simulink model "system2020b"  (R2020b)
settings: Solver=VariableStepAuto  StartTime=0.0  StopTime=50  RelTol=1e-3
InitFcn:
  | parametriEgo
values from neighbouring files (symbols this model uses):
  campnormalized = campmag/sqrt(campmag(1)^2+campmag(2)^2+campmag(3)^2)    [parametriEgo.m]
  g = 9.81    [kalman_jacobian.m]    (also in parametriEgo.m = [0; 0; -9.81])
  initial_conditions = [0,0,0*pi/180,0*pi/180,0,0]    [parametriEgo.m]
  k_e_qf = 0.1    [ego_control_gains_sensors.m]
  ki_e_nu_speed = 2.5    [ego_control_gains_sensors.m]
  kp_e_nu_phidot = 7    [ego_control_gains_sensors.m]
  kp_e_nu_speed = 6    [ego_control_gains_sensors.m]
  kp_e_nu_thetadot = 7    [ego_control_gains_sensors.m]
  kp_e_theta = 40    [ego_control_gains_sensors.m]
  l = 0.248    [parametriEgo.m]
  L = 0.379    [parametriEgo.m]
  mb = 21.7+0.536*10+0.381*2    (= 27.822)    [parametriEgo.m]
  mw = 1.6    [parametriEgo.m]
  P0 = 1500*eye(7)    [parametriEgo.m]
  r = 0.13    [parametriEgo.m]
  seedAcc1 = ceil(rand()*10)    [parametriEgo.m]
  seedAcc2 = ceil(rand()*10)    [parametriEgo.m]
  seedGyro1 = ceil(rand()*10)    [parametriEgo.m]
  seedGyro2 = ceil(rand()*10)    [parametriEgo.m]
  tau_max = 11    [parametriEgo.m]
  totAccNoisePower = (accNoiseDens* 10^-6 * 9.8)^2    (= 8.6436e-06)    [parametriEgo.m]
  totGyroNoisePower = (gyroNoiseDens * pi/180)^2    (= 3.04617419787e-06)    [parametriEgo.m]
  Ts = 1/100    (= 0.01)    [parametriEgo.m]
  TsController = 1/100    (= 0.01)    [parametriEgo.m]
  TsGraph = 1/100    (= 0.01)    [parametriEgo.m]
  x0 = zeros(7,1)    [parametriEgo.m]
undefined symbols (not defined in the file or in its folder): alpha
libraries: simulink_extras x45, simulink x10, eeGeneralControl x3
(part 2 of 3)

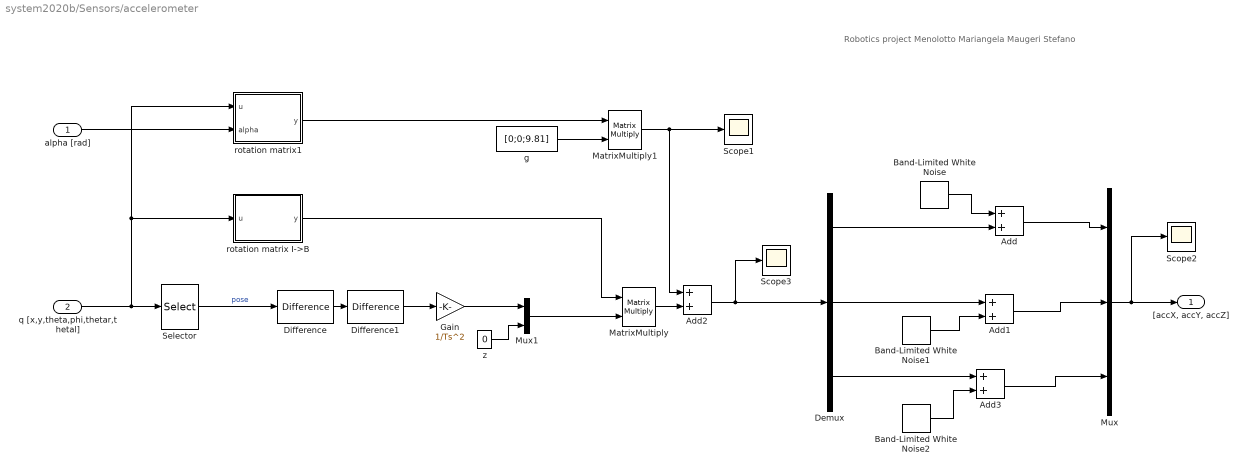
== system system2020b/Sensors/accelerometer ==
  note: Robotics project
      | Menolotto Mariangela
      | Maugeri Stefano
  alpha [rad] : Inport
  q [x,y,theta,phi,thetar,thetal] : Inport  Port=2
  Add{,1..3} (4 alike) : Sum
  Band-Limited White Noise : simulink/Sources/Band-Limited White Noise  Cov=abs(totAccNoisePower)  Ts=0.1  seed=abs(seedAcc1)+1
  Band-Limited White Noise1 : simulink/Sources/Band-Limited White Noise  Cov=totAccNoisePower  Ts=0.1  seed=abs(seedAcc2)+22
  Band-Limited White Noise2 : simulink/Sources/Band-Limited White Noise  Cov=totAccNoisePower  Ts=0.1  seed=abs(seedAcc1+13)
  Demux : Demux  Outputs=3
  Difference : simulink/Discrete/Difference  ICPrevInput=0.0  OutMin=[]  OutMax=[]  OutDataType=fixdt(1, 16)  OutScaling=2^-10  DoSatur=off
  Difference1 : simulink/Discrete/Difference  ICPrevInput=0.0  OutMin=[]  OutMax=[]  OutDataType=fixdt(1, 16)  OutScaling=2^-10  DoSatur=off
  Gain : Gain  Gain=1/Ts^2
  MatrixMultiply : Product  Multiplication=Matrix(*)
  MatrixMultiply1 : Product  Multiplication=Matrix(*)
  Mux : Mux  Inputs=3
  Mux1 : Mux  Inputs=2
  Scope1 : Scope
  Scope2 : Scope
  Scope3 : Scope
  Selector : Selector  InputPortWidth=6  IndexOptions=Index vector (dialog)  Indices=[1 2]  OutputSizes=1
  g : Constant  Value=[0;0;9.81]
  rotation matrix I->B : MATLAB Function  TreatAsAtomicUnit=on
  rotation matrix1 : MATLAB Function  TreatAsAtomicUnit=on
  z : Constant  Value=0
  "[accX, accY, accZ]" : Outport
  wires:
  q [x,y,theta,phi,thetar,thetal]/1 -> rotation matrix I->B/1(u), rotation matrix1/1(u), Selector/1
  Selector/1 -> Difference/1  "pose"
  Demux/1 -> Add/2
  Demux/2 -> Add1/1
  Band-Limited White Noise1/1 -> Add1/2
  Band-Limited White Noise/1 -> Add/1
  Mux/1 -> Scope2/1, "[accX, accY, accZ]"/1
  Add1/1 -> Mux/2
  Add/1 -> Mux/1
  z/1 -> Mux1/2
  Mux1/1 -> MatrixMultiply/2
  rotation matrix I->B/1(y) -> MatrixMultiply/1
  MatrixMultiply/1 -> Add2/2
  rotation matrix1/1(y) -> MatrixMultiply1/1
  g/1 -> MatrixMultiply1/2
  Add2/1 -> Scope3/1, Demux/1
  MatrixMultiply1/1 -> Add2/1, Scope1/1
  Demux/3 -> Add3/1
  Band-Limited White Noise2/1 -> Add3/2
  Add3/1 -> Mux/3
  alpha [rad]/1 -> rotation matrix1/2(alpha)
  Difference/1 -> Difference1/1
  Difference1/1 -> Gain/1
  Gain/1 -> Mux1/1

== system system2020b/Sensors/encoder ==
  note: Robotics project
      | Menolotto Mariangela
      | Maugeri Stefano
  q [x,y,theta,phi,thetar,thetal] : Inport
  Demux : Demux  Outputs=2
  Mux : Mux  Inputs=2
  Random Number : RandomNumber  Variance=0.03/3  SampleTime=0.1
  Random Number1 : RandomNumber  Variance=0.03/3  SampleTime=0.1
  Selector : Selector  InputPortWidth=6  IndexOptions=Index vector (dialog)  Indices=[5 6]  OutputSizes=1
  Sum : Sum  Inputs=++|
  Sum1 : Sum  Inputs=|++
  "thetar, thetal" : Outport
  wires:
  q [x,y,theta,phi,thetar,thetal]/1 -> Selector/1
  Selector/1 -> Demux/1
  Mux/1 -> "thetar, thetal"/1
  Sum/1 -> Mux/1
  Demux/1 -> Sum/2
  Sum1/1 -> Mux/2
  Demux/2 -> Sum1/1
  Random Number1/1 -> ?
  Random Number/1 -> ?

== system system2020b/Sensors/gyroscope ==
  note: Robotics project
      | Menolotto Mariangela
      | Maugeri Stefano
  "nu [v_avaz, theta dot, phi dot]" : Inport
  q [x,y,theta,phi,thetar,thetal] : Inport  Port=2
  Add : Sum
  Add1 : Sum
  Add2 : Sum
  Band-Limited White Noise : simulink/Sources/Band-Limited White Noise  Cov=totGyroNoisePower  Ts=0.1  seed=seedGyro1
  Band-Limited White Noise1 : simulink/Sources/Band-Limited White Noise  Cov=totGyroNoisePower  Ts=0.1  seed=seedGyro2+1
  Band-Limited White Noise2 : simulink/Sources/Band-Limited White Noise  Cov=totGyroNoisePower  Ts=0.1  seed=seedGyro1-2
  Demux : Demux  Outputs=3
  MATLAB Function : MATLAB Function  TreatAsAtomicUnit=on
  Mux : Mux  Inputs=3
  Radians to Degrees : simulink_extras/Transformations/Radians to Degrees
  Scope : Scope
  Scope1 : Scope
  Selector : Selector  InputPortWidth=3  IndexOptions=Index vector (dialog)  Indices=[2 3]  OutputSizes=1
  omega_c hat : Outport
  wires:
  "nu [v_avaz, theta dot, phi dot]"/1 -> Selector/1
  Selector/1 -> MATLAB Function/1(u)  "theta dot, phi dot"
  Demux/1 -> Add/2
  Demux/3 -> Add1/1
  Mux/1 -> Scope/1, omega_c hat/1
  Band-Limited White Noise/1 -> Add/1
  Band-Limited White Noise1/1 -> Add1/2
  Add/1 -> Mux/1
  Add1/1 -> Mux/3
  Add2/1 -> Mux/2
  MATLAB Function/1(omegac) -> Radians to Degrees/1, Demux/1
  q [x,y,theta,phi,thetar,thetal]/1 -> MATLAB Function/2(q)
  Demux/2 -> Add2/2
  Band-Limited White Noise2/1 -> Add2/1
  Radians to Degrees/1 -> Scope1/1

== system system2020b/Sensors/magnetometer    ==
  note: Robotics project
      | Menolotto Mariangela
      | Maugeri Stefano
  alpha [rad] : Inport
  q [x,y,theta,phi,thetar,thetal] : Inport  Port=2
  Add : Sum
  Band-Limited White Noise : simulink/Sources/Band-Limited White Noise  Cov=abs(totGyroNoisePower)  Ts=0.1  seed=seedGyro1
  MATLAB Function : MATLAB Function  TreatAsAtomicUnit=on
  magnetometer : Outport
  wires:
  MATLAB Function/1(y) -> Add/2
  alpha [rad]/1 -> MATLAB Function/1(alpha)
  q [x,y,theta,phi,thetar,thetal]/1 -> MATLAB Function/2(q)
  Band-Limited White Noise/1 -> Add/1
  Add/1 -> magnetometer/1

== system system2020b/Sensors/mux signals ==
  note: Robotics project
      | Menolotto Mariangela
      | Maugeri Stefano
  q [x,y,theta,phi,thetar,thetal] : Inport
  "nu [v_avaz, theta dot, phi dot]" : Inport  Port=2
  q_dot : Inport  Port=3
  Mux : Mux  Inputs=3
  "[q;nu]" : Outport
  wires:
  q [x,y,theta,phi,thetar,thetal]/1 -> Mux/1
  "nu [v_avaz, theta dot, phi dot]"/1 -> Mux/2
  Mux/1 -> "[q;nu]"/1
  q_dot/1 -> Mux/3

== system system2020b/Sensors/range finder ==
  note: Robotics project
      | Menolotto Mariangela
      | Maugeri Stefano
  q : Inport
  MATLAB Function1 : MATLAB Function  TreatAsAtomicUnit=on
  Quantizer : Quantizer  QuantizationInterval=0.001
  Quantizer1 : Quantizer  QuantizationInterval=0.001
  Random Number : RandomNumber  Variance=0.0000001  SampleTime=1/10
  Scope : Scope  NumInputPorts=2
  Scope1 : Scope
  Sum : Sum  Inputs=|++
  distance from ground : Outport
  wires:
  q/1 -> MATLAB Function1/1(q)  "[x,y,theta,phi,thetar,thetal]"
  MATLAB Function1/1(d) -> Scope/1, Sum/1  "new"
  Random Number/1 -> Sum/2, Scope1/1
  Sum/1 -> Quantizer/1, Quantizer1/1
  Quantizer/1 -> Scope/2
  Quantizer1/1 -> distance from ground/1

== system system2020b/Filtering/Kalman filter/store on workspace ==
  note: Robotics project
      | Menolotto Mariangela
      | Maugeri Stefano
  "[v_avanz real, thetadot, phidot] est" : Inport
  "[alpha, theta, phi] est" : Inport  Port=2
  Demux : Demux  Outputs=3
  Demux1 : Demux  Outputs=3
  Radians to Degrees : simulink_extras/Transformations/Radians to Degrees
  Radians to Degrees1 : simulink_extras/Transformations/Radians to Degrees
  Terminator : Terminator
  To Workspace : ToWorkspace  VariableName=thetadot_esimt_kalman  SaveFormat=Timeseries  SampleTime=TsGraph
  To Workspace1 : ToWorkspace  VariableName=phidot_esimt_kamlan  SaveFormat=Timeseries  SampleTime=TsGraph
  To Workspace2 : ToWorkspace  VariableName=alpha_esimt_kalman  SaveFormat=Timeseries  SampleTime=TsGraph
  To Workspace3 : ToWorkspace  VariableName=theta_esimt_kalman  SaveFormat=Timeseries  SampleTime=TsGraph
  To Workspace4 : ToWorkspace  VariableName=phi_esimt_kalman  SaveFormat=Timeseries  SampleTime=TsGraph
  wires:
  "[v_avanz real, thetadot, phidot] est"/1 -> Radians to Degrees/1
  "[alpha, theta, phi] est"/1 -> Radians to Degrees1/1
  Demux/1 -> Terminator/1
  Demux/2 -> To Workspace/1
  Demux/3 -> To Workspace1/1
  Demux1/1 -> To Workspace2/1
  Demux1/2 -> To Workspace3/1
  Demux1/3 -> To Workspace4/1
  Radians to Degrees/1 -> Demux/1
  Radians to Degrees1/1 -> Demux1/1

== system system2020b/Filtering/Mahony + distance sensor/mahony  with quaternions ==
  note: [v_avanz real, thetadot, phidot] est
  note: Robotics project
      | Menolotto Mariangela
      | Maugeri Stefano
  alpha real [rad] : Inport
  distance from ground : Inport  Port=2
  magnetometro : Inport  Port=3
  "[accX, accY, accZ] with noise" : Inport  Port=4
  omega_c hat with noise : Inport  Port=5
  "[q; nu; q_dot] real" : Inport  Port=6
  MATLAB Function : MATLAB Function  TreatAsAtomicUnit=on
  Manual Switch : ManualSwitch  CurrentSetting=0
  Mux1 : Mux  Inputs=3
  Radians to Degrees : simulink_extras/Transformations/Radians to Degrees
  Scope : Scope
  Selector : Selector  InputPortWidth=3  IndexOptions=Index vector (dialog)  Indices=3  OutputSizes=1
  Zero-Order Hold1 : ZeroOrderHold  SampleTime=Ts
  get phi : MATLAB Function  Commented=on  TreatAsAtomicUnit=on
  get phi1 : MATLAB Function  TreatAsAtomicUnit=on
  mahony filter qith quat : Subsystem
  mux signals : Subsystem
  scope differences (mahony) con quaternioni : Subsystem
  nu est : Outport
  "[q;nu] real" : Outport  Port=2
  "[alpha, theta, phi] est" : Outport  Port=3
  wires:
  "[accX, accY, accZ] with noise"/1 -> mahony filter qith quat/2("[accX, accY, accZ]")
  "[q; nu; q_dot] real"/1 -> mux signals/1("[q; nu; q_dot] real")
  Mux1/1 -> Zero-Order Hold1/1
  omega_c hat with noise/1 -> MATLAB Function/1(omega_c), mahony filter qith quat/3(omega_c hat with noise)
  magnetometro/1 -> mahony filter qith quat/4(magnetometro)
  mux signals/2("[q;nu]") -> "[q;nu] real"/1, scope differences (mahony) con quaternioni/3("[q;nu] real")
  alpha real [rad]/1 -> scope differences (mahony) con quaternioni/4(real alpha)
  get phi/1(phi_star) -> Manual Switch/1
  MATLAB Function/1(thetadot) -> Mux1/2  "theta dot"
  MATLAB Function/2(phidot) -> Mux1/3
  Zero-Order Hold1/1 -> nu est/1, scope differences (mahony) con quaternioni/1(nu est)
  mahony filter qith quat/1("[alpha, theta, phi] est") -> scope differences (mahony) con quaternioni/2("[alpha, theta, phi] est"), "[alpha, theta, phi] est"/1, Selector/1  "[alpha theta phi] est"
  Selector/1 -> MATLAB Function/2(phi)  "phi"
  mux signals/1(v_avanz) -> Mux1/1
  distance from ground/1 -> get phi/1(d), get phi1/1(d)
  Manual Switch/1 -> Radians to Degrees/1, mahony filter qith quat/1(phi_star)
  get phi1/1(phi_star) -> Manual Switch/2
  Radians to Degrees/1 -> Scope/1

== system system2020b/Filtering/Mahony + distance sensor/mahony filter ==
  note: Robotics project
      | Menolotto Mariangela
      | Maugeri Stefano
  phi_star : Inport
  "[accX, accY, accZ]" : Inport  Port=2
  omega_c hat with noise : Inport  Port=3
  magnetometro : Inport  Port=4
  Clock : Clock
  Delay : Delay  DelayLength=1  InitialCondition=eye(3)  SampleTime=Ts
  Delay1 : Delay  DelayLength=1  InitialCondition=[0;0;0]  SampleTime=Ts
  Delay2 : Delay  DelayLength=1  SampleTime=Ts
  MATLAB Function : MATLAB Function  TreatAsAtomicUnit=on
  Mux2 : Mux  Inputs=3
  Zero-Order Hold4 : ZeroOrderHold  SampleTime=Ts
  "get angles " : MATLAB Function  TreatAsAtomicUnit=on
  "[alpha, theta, phi] est" : Outport
  wires:
  MATLAB Function/1(R) -> "get angles "/1(R), Delay/1  "R"
  Delay/1 -> MATLAB Function/4(Rprev)
  MATLAB Function/2(I) -> Delay1/1
  Delay1/1 -> MATLAB Function/5(Iprev)
  "[accX, accY, accZ]"/1 -> MATLAB Function/1(acc)
  omega_c hat with noise/1 -> MATLAB Function/2(gyro)
  magnetometro/1 -> MATLAB Function/3(mb)
  phi_star/1 -> "get angles "/2(phi_star)
  "get angles "/1(alpha) -> Mux2/1
  "get angles "/3(phi) -> Mux2/3
  "get angles "/2(theta) -> Delay2/1, Mux2/2
  Delay2/1 -> "get angles "/4(old_theta)
  Mux2/1 -> "[alpha, theta, phi] est"/1  "angles est"
  Clock/1 -> Zero-Order Hold4/1
  Zero-Order Hold4/1 -> "get angles "/3(t)

== system system2020b/Filtering/Mahony + distance sensor/store on workspace ==
  note: Robotics project
      | Menolotto Mariangela
      | Maugeri Stefano
  "[v_avanz real, thetadot, phidot] est" : Inport
  "[alpha, theta, phi] est" : Inport  Port=2
  Demux : Demux  Outputs=3
  Demux1 : Demux  Outputs=3
  Radians to Degrees : simulink_extras/Transformations/Radians to Degrees
  Radians to Degrees1 : simulink_extras/Transformations/Radians to Degrees
  Terminator : Terminator
  To Workspace : ToWorkspace  VariableName=thetadot_esimt_mahony  SaveFormat=Timeseries  SampleTime=TsGraph
  To Workspace1 : ToWorkspace  VariableName=phidot_esimt_mahony  SaveFormat=Timeseries  SampleTime=TsGraph
  To Workspace2 : ToWorkspace  VariableName=alpha_esimt_mahony  SaveFormat=Timeseries  SampleTime=TsGraph
  To Workspace3 : ToWorkspace  VariableName=theta_esimt_mahony  SaveFormat=Timeseries  SampleTime=TsGraph
  To Workspace4 : ToWorkspace  VariableName=phi_esimt_mahony  SaveFormat=Timeseries  SampleTime=TsGraph
  wires:
  "[v_avanz real, thetadot, phidot] est"/1 -> Radians to Degrees/1
  "[alpha, theta, phi] est"/1 -> Radians to Degrees1/1
  Demux/1 -> Terminator/1
  Demux/2 -> To Workspace/1
  Demux/3 -> To Workspace1/1
  Demux1/1 -> To Workspace2/1
  Demux1/2 -> To Workspace3/1
  Demux1/3 -> To Workspace4/1
  Radians to Degrees/1 -> Demux/1
  Radians to Degrees1/1 -> Demux1/1

== system system2020b/Physical system/old model/LQR con linearizzato ==
  note: Robotics project
      | Menolotto Mariangela
      | Maugeri Stefano
  q : Inport
  nu : Inport  Port=2
  Gain : Gain  Gain=-1
  Integrator : Integrator
  LQR : MATLAB Function  TreatAsAtomicUnit=on
  MATLAB Function1 : MATLAB Function  TreatAsAtomicUnit=on
  MATLAB Function2 : MATLAB Function  TreatAsAtomicUnit=on
  MatrixMultiply : Product  Multiplication=Matrix(*)
  Mux : Mux  Inputs=3
  Saturation : Saturate  UpperLimit=tau_max  LowerLimit=-tau_max
  Selector : Selector  InputPortWidth=6  IndexOptions=Index vector (dialog)  Indices=[3 4]  OutputSizes=1
  Selector1 : Selector  InputPortWidth=3  IndexOptions=Index vector (dialog)  Indices=1  OutputSizes=1
  To Workspace1 : ToWorkspace  VariableName=nu1_int  SaveFormat=Timeseries  SampleTime=TsGraph
  tau : Outport
  wires:
  MATLAB Function1/1(B_ss_numerica) -> LQR/2(B_ss)
  LQR/1(K) -> Gain/1
  MATLAB Function2/1(A_ss_numerica) -> LQR/1(A_ss)
  Gain/1 -> MatrixMultiply/1
  MatrixMultiply/1 -> Saturation/1  "u = - Kx"
  nu/1 -> Selector1/1, Mux/1
  q/1 -> Selector/1
  Mux/1 -> MatrixMultiply/2
  Selector/1 -> Mux/3
  Saturation/1 -> tau/1  "nu"
  Selector1/1 -> Integrator/1
  Integrator/1 -> Mux/2, To Workspace1/1

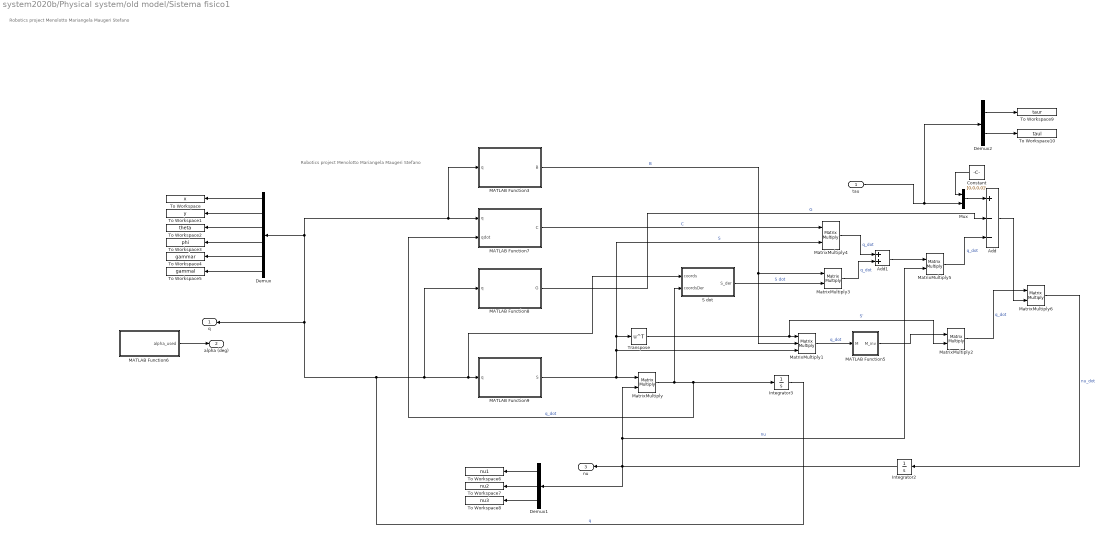
== system system2020b/Physical system/old model/Sistema fisico1 ==
  note: Robotics project
      | Menolotto Mariangela
      | Maugeri Stefano
  note: Robotics project
      | Menolotto Mariangela
      | Maugeri Stefano
  tau : Inport
  Add : Sum  Inputs=+--
  Add1 : Sum
  Constant : Constant  Value=[0,0,0,0]'
  Demux : Demux  Outputs=6
  Demux1 : Demux  Outputs=3
  Demux2 : Demux  Outputs=2
  Integrator2 : Integrator  InitialCondition=[0; 0; 0]
  Integrator3 : Integrator  InitialCondition=initial_conditions
  MATLAB Function3 : MATLAB Function  TreatAsAtomicUnit=on
  MATLAB Function5 : MATLAB Function  TreatAsAtomicUnit=on
  MATLAB Function6 : MATLAB Function  TreatAsAtomicUnit=on
  MATLAB Function7 : MATLAB Function  TreatAsAtomicUnit=on
  MATLAB Function8 : MATLAB Function  TreatAsAtomicUnit=on
  MATLAB Function9 : MATLAB Function  TreatAsAtomicUnit=on
  MatrixMultiply{,2..6} (6 alike) : Product  Multiplication=Matrix(*)
  MatrixMultiply1 : Product  Inputs=3  Multiplication=Matrix(*)
  Mux : Mux  Inputs=2
  S dot : MATLAB Function  TreatAsAtomicUnit=on
  To Workspace : ToWorkspace  VariableName=x  SaveFormat=Timeseries  SampleTime=TsGraph
  To Workspace1 : ToWorkspace  VariableName=y  SaveFormat=Timeseries  SampleTime=TsGraph
  To Workspace10 : ToWorkspace  VariableName=taul  SaveFormat=Timeseries  SampleTime=TsGraph
  To Workspace2 : ToWorkspace  VariableName=theta  SaveFormat=Timeseries  SampleTime=TsGraph
  To Workspace3 : ToWorkspace  VariableName=phi  SaveFormat=Timeseries  SampleTime=TsGraph
  To Workspace4 : ToWorkspace  VariableName=gammar  SaveFormat=Timeseries  SampleTime=TsGraph
  To Workspace5 : ToWorkspace  VariableName=gammal  SaveFormat=Timeseries  SampleTime=TsGraph
  To Workspace6 : ToWorkspace  VariableName=nu1  SaveFormat=Timeseries  SampleTime=TsGraph
  To Workspace7 : ToWorkspace  VariableName=nu2  SaveFormat=Timeseries  SampleTime=TsGraph
  To Workspace8 : ToWorkspace  VariableName=nu3  SaveFormat=Timeseries  SampleTime=TsGraph
  To Workspace9 : ToWorkspace  VariableName=taur  SaveFormat=Timeseries  SampleTime=TsGraph
  Transpose : Math  Operator=transpose  SaturateOnIntegerOverflow=on
  q : Outport
  alpha (deg) : Outport  Port=2
  nu : Outport  Port=3
  wires:
  MATLAB Function9/1(S) -> MatrixMultiply1/3, Transpose/1, MatrixMultiply4/2, MatrixMultiply/1  "S"
  Integrator3/1 -> MATLAB Function3/1(q), MATLAB Function7/1(q), Demux/1, q/1, MATLAB Function8/1(q), MATLAB Function9/1(q), S dot/1(coords)  "q"
  S dot/1(S_der) -> MatrixMultiply3/2  "S dot"
  MATLAB Function3/1(B) -> MatrixMultiply3/1, MatrixMultiply1/2  "B"
  Integrator2/1 -> Demux1/1, MatrixMultiply5/2, MatrixMultiply/2, nu/1  "nu"
  MATLAB Function8/1(G) -> Add/2  "G"
  Transpose/1 -> MatrixMultiply2/2, MatrixMultiply1/1  "S'"
  MatrixMultiply1/1 -> MATLAB Function5/1(M)  "q_dot"
  MatrixMultiply3/1 -> Add1/2  "q_dot"
  MatrixMultiply/1 -> MATLAB Function7/2(qdot), Integrator3/1, S dot/2(coordsDer)  "q_dot"
  MATLAB Function7/1(C) -> MatrixMultiply4/1  "C"
  Add1/1 -> MatrixMultiply5/1
  MatrixMultiply4/1 -> Add1/1  "q_dot"
  MatrixMultiply5/1 -> Add/3  "q_dot"
  Add/1 -> MatrixMultiply6/2
  MatrixMultiply6/1 -> Integrator2/1  "nu_dot"
  MATLAB Function5/1(M_inv) -> MatrixMultiply2/1
  MatrixMultiply2/1 -> MatrixMultiply6/1  "q_dot"
  MATLAB Function6/1(alpha_used) -> alpha (deg)/1
  Demux/5 -> To Workspace4/1
  Demux/2 -> To Workspace1/1
  Demux/1 -> To Workspace/1
  Demux/3 -> To Workspace2/1
  Demux/4 -> To Workspace3/1
  Demux/6 -> To Workspace5/1
  Mux/1 -> Add/1
  Constant/1 -> Mux/1
  Demux1/1 -> To Workspace6/1
  Demux1/2 -> To Workspace7/1
  Demux1/3 -> To Workspace8/1
  tau/1 -> Demux2/1, Mux/2
  Demux2/1 -> To Workspace9/1
  Demux2/2 -> To Workspace10/1

== system system2020b/Filtering/Mahony + distance sensor/mahony  with quaternions/mahony filter qith quat ==
  note: Robotics project
      | Menolotto Mariangela
      | Maugeri Stefano
  phi_star : Inport
  "[accX, accY, accZ]" : Inport  Port=2
  omega_c hat with noise : Inport  Port=3
  magnetometro : Inport  Port=4
  Delay : Delay  DelayLength=1  InitialCondition=[1;0;0;0]  SampleTime=Ts
  Delay1 : Delay  DelayLength=1  InitialCondition=[0;0;0]  SampleTime=Ts
  MATLAB Function : MATLAB Function  TreatAsAtomicUnit=on
  Mux2 : Mux  Inputs=3
  Radians to Degrees : simulink_extras/Transformations/Radians to Degrees
  Scope : Scope
  get angles : MATLAB Function  TreatAsAtomicUnit=on
  "[alpha, theta, phi] est" : Outport
  wires:
  MATLAB Function/1(q) -> get angles/1(q), Delay/1  "R"
  Delay/1 -> MATLAB Function/4("q ")
  MATLAB Function/2(I) -> Delay1/1
  Delay1/1 -> MATLAB Function/5(Iprev)
  "[accX, accY, accZ]"/1 -> MATLAB Function/1(acc)
  omega_c hat with noise/1 -> MATLAB Function/2(gyro)
  magnetometro/1 -> MATLAB Function/3(mb)
  phi_star/1 -> get angles/2(phi_star)
  get angles/1(alpha) -> Mux2/1
  get angles/2(theta) -> Mux2/2
  get angles/3(phi) -> Mux2/3
  Mux2/1 -> "[alpha, theta, phi] est"/1, Radians to Degrees/1  "angles est"
  Radians to Degrees/1 -> Scope/1

== system system2020b/Filtering/Mahony + distance sensor/mahony  with quaternions/mux signals ==
  note: Robotics project
      | Menolotto Mariangela
      | Maugeri Stefano
  "[q; nu; q_dot] real" : Inport
  Selector : Selector  InputPortWidth=15  IndexOptions=Index vector (dialog)  Indices=7  OutputSizes=1
  Selector1 : Selector  InputPortWidth=15  IndexOptions=Index vector (dialog)  Indices=[1:9]  OutputSizes=1
  v_avanz : Outport
  "[q;nu]" : Outport  Port=2
  wires:
  "[q; nu; q_dot] real"/1 -> Selector1/1, Selector/1
  Selector/1 -> v_avanz/1  "v_avanz"
  Selector1/1 -> "[q;nu]"/1  "[q;nu]"

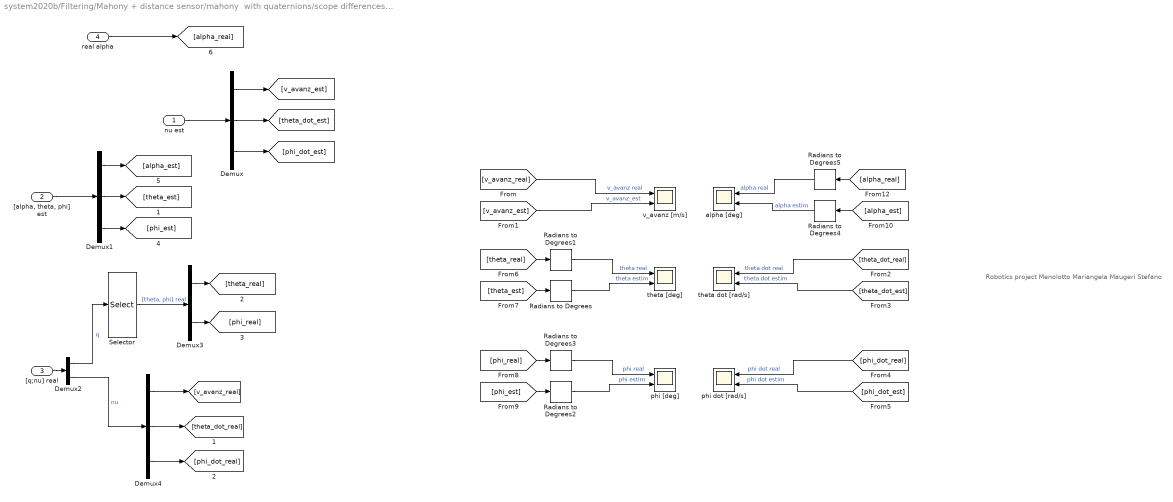
== system system2020b/Filtering/Mahony + distance sensor/mahony  with quaternions/scope differences (mahony) con quaternioni ==
  note: Robotics project
      | Menolotto Mariangela
      | Maugeri Stefano
  nu est : Inport
  "[alpha, theta, phi] est" : Inport  Port=2
  "[q;nu] real" : Inport  Port=3
  real alpha : Inport  Port=4
  Demux : Demux  Outputs=3
  Demux1 : Demux  Outputs=3
  Demux2 : Demux  Outputs=[6,3]
  Demux3 : Demux  Outputs=2
  Demux4 : Demux  Outputs=3
  Radians to Degrees{,1..5} (6 alike) : simulink_extras/Transformations/Radians to Degrees
  Selector : Selector  InputPortWidth=6  IndexOptions=Index vector (dialog)  Indices=[3 4]  OutputSizes=1
  alpha [deg] : Scope  NumInputPorts=2
  phi [deg] : Scope  NumInputPorts=2
  phi dot [rad/s] : Scope  NumInputPorts=2
  theta [deg] : Scope  NumInputPorts=2
  theta dot [rad/s] : Scope  NumInputPorts=2
  v_avanz [m/s] : Scope  NumInputPorts=2
  wires:
  nu est/1 -> Demux/1
  "[alpha, theta, phi] est"/1 -> Demux1/1
  "[q;nu] real"/1 -> Demux2/1
  Demux2/1 -> Selector/1  "q"
  Selector/1 -> Demux3/1  "[theta, phi] real"
  Demux2/2 -> Demux4/1  "nu"
  Demux4/1 -> [v_avanz_real]
  [v_avanz_real] -> v_avanz [m/s]/1  "v_avanz real"
  Demux/1 -> [v_avanz_est]
  [v_avanz_est] -> v_avanz [m/s]/2  "v_avanz_est"
  [theta_dot_real] -> theta dot [rad/s]/1  "theta dot real"
  [theta_dot_est] -> theta dot [rad/s]/2  "theta dot estim"
  [phi_dot_real] -> phi dot [rad/s]/1  "phi dot real"
  [phi_dot_est] -> phi dot [rad/s]/2  "phi dot estim"
  Demux/2 -> [theta_dot_est]
  Demux/3 -> [phi_dot_est]
  Demux4/2 -> [theta_dot_real]
  Demux4/3 -> [phi_dot_real]
  [theta_est] -> Radians to Degrees/1
  [theta_real] -> Radians to Degrees1/1
  Radians to Degrees/1 -> theta [deg]/2  "theta estim"
  Radians to Degrees1/1 -> theta [deg]/1  "theta real"
  Demux1/2 -> [theta_est]
  Demux3/1 -> [theta_real]
  Radians to Degrees3/1 -> phi [deg]/1  "phi real"
  [phi_real] -> Radians to Degrees3/1
  [phi_est] -> Radians to Degrees2/1
  Radians to Degrees2/1 -> phi [deg]/2  "phi estim"
  Demux3/2 -> [phi_real]
  Demux1/3 -> [phi_est]
  Demux1/1 -> [alpha_est]
  real alpha/1 -> [alpha_real]
  Radians to Degrees4/1 -> alpha [deg]/2  "alpha estim"
  [alpha_real] -> Radians to Degrees5/1
  Radians to Degrees5/1 -> alpha [deg]/1  "alpha real"
  [alpha_est] -> Radians to Degrees4/1

== matlab function system2020b/Filtering/Mahony + distance sensor/get phi from distance sensor ==
  data: d input; phi_star output; r parameter
function phi_star = fcn(d, r)
% Robotics project, Menolotto Mariangela & Stefano Maugeri


phi_star = asin((d^2-r^2)/(d^2+r^2));

== matlab function system2020b/Sensors/gyroscope/MATLAB Function ==
  data: u input; omegac output; q input
function omegac = fcn(u, q)
% Robotics project, Menolotto Mariangela & Stefano Maugeri

phi = q(4);

thetadot = u(1);
phidot = u(2);

Rphi = [1, 0, 0; 0, cos(phi), -sin(phi); 0, sin(phi), cos(phi)] ;


omegac = [phidot, 0, 0]'+ Rphi'*[0,0,thetadot]';

== matlab function system2020b/Filtering/Mahony + distance sensor/MATLAB Function ==
  data: omega_c input; thetadot output; phidot output; phi input
function [thetadot, phidot] = fcn(omega_c, phi)
% Robotics project, Menolotto Mariangela & Stefano Maugeri
% get phidot e thetadot from gyro

phidot = omega_c(1);


thetadot = real(omega_c(3)/cos(complex(phi)));
%thetadot = omega_c(2)/(acos((phi)));

== matlab function system2020b/Physical system/old model/LQR con linearizzato/MATLAB Function1 ==
  data: B_ss_numerica output
function B_ss_numerica = B_ss_num()

%theta= pi/2;
theta= 0;
phi = 0;
%phi = -alpha;

B_ss_numerica=B_ss_file(phi,theta);

== matlab function system2020b/Filtering/Mahony + distance sensor/mahony  with quaternions/MATLAB Function ==
  data: omega_c input; thetadot output; phidot output; phi input
% Robotics project, Menolotto Mariangela & Stefano Maugeri
function [thetadot, phidot] = fcn(omega_c, phi)
% get phidot e thetadot from gyro

phidot = omega_c(1);


thetadot = real(omega_c(3)/acos(complex(phi)));
%thetadot = omega_c(2)/(acos((phi)));

== matlab function system2020b/Physical system/old model/LQR con linearizzato/MATLAB Function2 ==
  data: A_ss_numerica output
function A_ss_numerica = A_ss_num()

%theta= pi/2;
theta= 0;
%phi = -alpha;
phi = 0;

thetadot = 0;
phidot = 0;

nu1 = 0;
nu2 = 0;
nu3 = 0;
taul=0;
taur=0;

A_ss_numerica=A_ss_file(alpha,nu1,nu2,nu3,phi,taul,taur,theta);

== matlab function system2020b/Filtering/Mahony + distance sensor/mahony  with quaternions/get phi ==
  data: d input; phi_star output; r parameter
% Robotics project, Menolotto Mariangela & Stefano Maugeri
function phi_star = fcn(d, r)



phi_star = -atan2(sqrt(d^2-r^2), r);

== matlab function system2020b/Filtering/Mahony + distance sensor/mahony  with quaternions/get phi1 ==
  data: d input; phi_star output; r parameter
% Robotics project, Menolotto Mariangela & Stefano Maugeri
function phi_star = fcn(d, r)


phi_star = asin((d^2-r^2)/(d^2+r^2));

== matlab function system2020b/Filtering/Mahony + distance sensor/mahony  with quaternions/mahony filter qith quat/MATLAB Function ==
  data: acc input; q output; gyro input; mb input; q input; I output; Iprev input; Ts parameter; campnormalized parameter
function [q, I] = fcn(acc, gyro, mb, q, Iprev, Ts, campnormalized)
% Robotics project, Menolotto Mariangela & Stefano Maugeri

dt = Ts;

%kp=4; oppure 6
%ki=1.2;
kp=3.5;
ki=1.3;
l_acc = 1; 
l_mag = 0.2;


mod_a = sqrt(acc(1)^2+acc(2)^2+acc(3)^2);

acc = acc/mod_a;
mb = mb/norm(mb);

g_b=q_prod(q_prod(conjugate(q),[0,0,0,-1]'), q);
m_b=q_prod(q_prod(conjugate(q),[0,campnormalized]'), q);

e_a = cross(acc, g_b(2:4));
e_m = cross(mb, m_b(2:4));

e = l_acc * e_a + l_mag * e_m;

I = Iprev + ki * e * dt;

deomega = kp*e + I;
    
omega = deomega + gyro;

%omegaSkew = [0, - omega(3), omega(2); omega(3), 0, -omega(1); -omega(2), omega(1), 0];

qe = q + 0.5 * q_prod(q, [0; omega])* dt;

norm_q = sqrt(q(1)*q(1) + q(2)*q(2) + q(3)*q(3) + q(4)*q(4));

q = qe/norm_q;

end

function q_con = conjugate(q)
    q_con = q;
    q_con(2) = -q(2);
    q_con(3) = -q(3);
    q_con(4) = -q(4);
end

function quad_prod = q_prod(p, q)
    quad_prod = q;
    quad_prod(1) = p(1)*q(1)-p(2)*q(2)-p(3)*q(3)-p(4)*q(4);
    quad_prod(2) = p(1)*q(2)+p(2)*q(1)+p(3)*q(4)-p(4)*q(3);
    quad_prod(3) = p(1)*q(3)-p(2)*q(4)+p(3)*q(1)+p(4)*q(2);
    quad_prod(4) = p(1)*q(4)+p(2)*q(3)-p(3)*q(2)+p(4)*q(1);    
end

== matlab function system2020b/Filtering/Mahony + distance sensor/mahony  with quaternions/mahony filter qith quat/get angles ==
  data: q input; alpha output; theta output; phi output; phi_star input
% Robotics project, Menolotto Mariangela & Stefano Maugeri
%% We are looking for [alpha, theta, phi] from q

function [alpha, theta, phi] = fcn(q, phi_star)
%     q0=q(1);
%     q1=q(2);
%     q2=q(3);
%     q3=q(4);
    
%     alpha = atan2(2*(q1*q3-q0*q2), 2*(q0*q3+q1*q2));
%     theta = atan2(sqrt(4*(q1*q3-q0*q2)^2 + 4*(q0*q3+q1*q2)^2), 2*(q0^2+q1^2-0.5));
%     phi = atan2(2*(q0*q2+q1*q3), 2*(q0*q3-q1*q2));
    coder.extrinsic('quat2angle');
    %coder.extrinsic('lqr')
    alpha = 0;
    theta = 0;
    phi=0;

    [angles_x, angles_y, angles_z] = quat2angle(q', 'XZX');

    alpha = angles_x(1);
    theta = angles_y(1);
    phi = angles_z(1);
end

== matlab function system2020b/Filtering/Mahony + distance sensor/mahony filter/get angles  ==
  data: R input; alpha output; theta output; phi output; phi_star input; t input; old_theta input
%% We are looking for [alpha, theta, phi] from R
% Robotics project, Menolotto Mariangela & Stefano Maugeri

function [alpha, theta, phi] = fcn(R, phi_star, t, old_theta)
%% This theta is right in module but not in sign because its module sqrt(a^2+b^2)

theta = atan2(sqrt(R(2,1)^2 + R(3,1)^2), R(1,1));
%             ^ + or -

%% Determinate sign
sign = 0;

if R(2, 1) > 0 && R(3,1) > 0
    if abs(theta) > 0 && abs(theta) < 180*pi/180
        sign = 1;
    else
        sign = -1;
    end
elseif R(2, 1) < 0 && R(3,1) < 0
    if abs(theta) > 0 && abs(theta) < 180*pi/180
        sign = -1;
    else
        sign = 1;
    end
elseif R(2, 1) > 0 && R(3,1) < 0
    if abs(theta) > 0 && abs(theta) < 180*pi/180
        sign = 1;
    else
        sign = -1;
    end
elseif R(2, 1) < 0 && R(3,1) > 0
    if abs(theta) > 0 && abs(theta) < 180*pi/180
        sign = -1;
    else
        sign = 1;
    end
elseif R(2, 1) == 0 && R(3,1) == 0
    fprintf("Err 1\n") % there are a lot of combinations
else
    fprintf("Err 2\n"); % it should never happen
end

theta = atan2(sign * sqrt(R(2,1)^2 + R(3,1)^2), R(1,1));
%               ^ its correct sign

%%




%% Resolve singularity


if abs(theta*180/pi) < 15
    alpha = atan2(R(3,2), R(2,2)) - phi_star;
    phi = phi_star;
elseif theta >= 178.3*pi/180 && theta <= 181.7*pi/180
%     alpha = - atan2(R(3,2), -R(2,2)) + phi_star;
    phi = - phi_star;
    alpha = - atan2(R(2,3), R(3, 3)) + phi;
    
% elseif old_theta <= -178.3*pi/180 && old_theta >= -181.7*pi/180
%     phi = -phi_star;
%     alpha = - atan2(R(2,3), R(3, 3)) + phi;

elseif theta > 0
     alpha = atan2(R(3,1), R(2,1));
     phi = atan2(R(1,3), -R(1,2)); 
else
     alpha = atan2(-R(3,1), -R(2,1));
     phi = atan2(-R(1,3), +R(1,2));
end

%%    

if old_theta >= 178 * pi/180 && theta < 0
    theta = theta + 2*pi;
       
elseif old_theta <= -178 * pi/180 && theta > 0
    theta = theta - 2*pi;
end
%elseif old_theta >= 358 * pi/180 && theta <


end

== matlab function system2020b/Physical system/old model/Sistema fisico1/MATLAB Function5 ==
  data: M input; M_inv output
function M_inv = inverse(M)

M_inv = inv(M);

== matlab function system2020b/Physical system/old model/Sistema fisico1/MATLAB Function6 ==
  data: alpha_used output; alpha parameter
function alpha_used = from_workspace(alpha)

alpha_used=alpha*180/pi;

== matlab function system2020b/Physical system/old model/Sistema fisico1/S dot ==
  data: coords input; S_der output; r parameter; coordsDer input
function S_der = matrix_S_der(coords,r, coordsDer)
% Robotics project, Menolotto Mariangela & Stefano Maugeri

theta = coords(3);
thetadot = coordsDer(3);

S_der = zeros(6,3);

S_der = [-cos(theta)*thetadot, 0, 0;
    -sin(theta)*thetadot, 0, 0;
    0, 0, 0;
    0, 0, 0;
    0, 0, 0;
    0, 0, 0];

== matlab function system2020b/Reference generator/ref 1, id 2/MATLAB Function ==
  data: time input; control_type output; v_avanz output; theta_ref output; alpha output
% Robotics project, Menolotto Mariangela & Stefano Maugeri
function [control_type, v_avanz, theta_ref, alpha] = fcn1(time)
% alpha = 0, theta=0, 1 gradino di velocità a 0.2 e un altro per fermarlo
%
speed = 1;              % speed controller
position = 2;           % return to zero controller

control_type = speed;   % could be 'speed' or 'position' 
v_avanz = 0;            % forward speed [m/s]
theta_ref = 0;          % theta target [deg]
alpha = 0;              % alpha [deg]

step = [10, 20, 30];

%% step 1
if time < step(1)
    v_avanz=0;
end

%% step 2
if (time>=step(1) && time < step(2))
    v_avanz=0.25;
end

%% step 3
if (time >= step(2) && time <= step(3))
    v_avanz=0;
end

== matlab function system2020b/Reference generator/ref 2, id 3/MATLAB Function ==
  data: time input; control_type output; v_avanz output; theta_ref output; alpha output
% Robotics project, Menolotto Mariangela & Stefano Maugeri
function [control_type, v_avanz, theta_ref, alpha] = fcn1(time)
% alpha = 0, theta=0, 1 gradino di velocità a 0.2 e un altro per fermarlo
%
speed = 1;              % speed controller
position = 2;           % return to zero controller

control_type = speed;   % could be 'speed' or 'position' 
v_avanz = 0;            % forward speed [m/s]
theta_ref = 0;          % theta target [deg]
alpha = 0;              % alpha [deg]

step = [10, 20, 30];

%% step 1
if time < step(1)
    v_avanz=0;
end

%% step 2
if (time>=step(1) && time < step(2))
    v_avanz=0.25;
    theta_ref = -90;
end

%% step 3
if (time >= step(2) && time <= step(3))
    v_avanz=0;
end

== matlab function system2020b/Reference generator/ref 4, id 5/MATLAB Function ==
  data: time input; control_type output; v_avanz output; theta_ref output; alpha output
% Robotics project, Menolotto Mariangela & Stefano Maugeri
function [control_type, v_avanz, theta_ref, alpha] = fcn3(time)
% alpha = 0, theta=0, 1 gradino di velocità a 0.2 e un altro per fermarlo
%
speed = 1;              % speed controller
position = 2;           % return to zero controller

control_type = speed;   % could be 'speed' or 'position' 
v_avanz = 0;            % forward speed [m/s]
theta_ref = 0;          % theta target [deg]
alpha = 0;              % alpha [deg]

step = [10, 20, 30, 40];

%% step 1
if time < step(1)
    v_avanz=0;
end

%% step 2
if (time>=step(1) && time < step(2))
    alpha = (time-step(1)) * 3;
    if alpha > 15 
        alpha = 15;
    end
    alpha = -alpha;
    theta_ref = 0;
end

%% step 3
if (time >= step(2) && time <= step(3))
    alpha = -15;
    theta_ref = 360;    
end


%% step 4
if (time >= step(3) && time <= step(4))
    theta_ref = 360;
    alpha = 15 - (time-step(3)) * 3;
    if alpha < 0 
        alpha = 0;
    end
    alpha = - alpha;

end
%% end

if time > step(4)
   theta_ref = 360;
   alpha = 0;
   v_ref = 0;
end

== matlab function system2020b/Controller/model/MATLAB Function1 ==
  data: angles input; S output; r parameter; l parameter
function S = matrix_S(angles, r, l)
% Robotics project, Menolotto Mariangela & Stefano Maugeri
%theta = q(3);
theta = angles(2);

S = [-sin(theta), 0, 0;
    cos(theta), 0, 0;
    0, 1, 0;
    0, 0, 1;
    -1/r, -l/r, -1;
    -1/r, l/r, -1];

== matlab function system2020b/Reference generator/ref 5, id 6/MATLAB Function ==
  data: time input; control_type output; v_avanz output; theta_ref output; alpha output
% Robotics project, Menolotto Mariangela & Stefano Maugeri
function [control_type, v_avanz, theta_ref, alpha] = fcn5(time)
% alpha = 0, theta=0, 1 gradino di velocità a 0.2 e un altro per fermarlo
%
speed = 1;              % speed controller
position = 2;           % return to zero controller

control_type = speed;   % could be 'speed' or 'position' 
v_avanz = 0;            % forward speed [m/s]
theta_ref = 0;          % theta target [deg]
alpha = 0;              % alpha [deg]

step = [10, 20, 30, 50];

%% step 1
if time < step(1)
    v_avanz=0;
end

%% step 2
if (time>=step(1) && time < step(2))
    alpha = (time-step(1)) * 3;
    if alpha > 20 
        alpha = 20;
    end
    alpha = -alpha;
end

%% step 3
if (time >= step(2) && time <= step(3))
    alpha = -20;
end


%% step 4
if (time >= step(3) && time <= step(4))
    alpha = 20 - (time-step(3)) * 3;
    if alpha < -20
        alpha = -20;
    end
    alpha = - alpha;
end

if time > step(4)
    alpha = 20;
end

== matlab function system2020b/Sensors/magnetometer   /MATLAB Function ==
  data: alpha input; y output; q input
function y = fcn(alpha, q)
% Robotics project, Menolotto Mariangela & Stefano Maugeri

%Earth's magnetic field strength, m_e,
% computed on: https://www.ngdc.noaa.gov/geomag/calculators/magcalc.shtml#igrfwmm

m_e = [0.238836 -0.010851 0.392423]'; 

theta = q(3);
phi = q(4);

Ralpha = [1, 0, 0; 0, cos(alpha), -sin(alpha); 0, sin(alpha), cos(alpha)];
Rtheta = [cos(theta), -sin(theta), 0; sin(theta), cos(theta), 0; 0, 0, 1];
Rphi = [1, 0, 0; 0, cos(phi), -sin(phi); 0, sin(phi), cos(phi)];


y = Rphi'*Rtheta' * Ralpha' * m_e;

== matlab function system2020b/Reference generator/ref 6, id 7/MATLAB Function ==
  data: time input; control_type output; v_avanz output; theta_ref output; alpha output
% Robotics project, Menolotto Mariangela & Stefano Maugeri
function [control_type, v_avanz, theta_ref, alpha] = fcn6(time)
% alpha = 0, theta=0, 1 gradino di velocità a 0.2 e un altro per fermarlo
%
speed = 1;              % speed controller
position = 2;           % return to zero controller

control_type = speed;   % could be 'speed' or 'position' 
v_avanz = 0.25;            % forward speed [m/s]
theta_ref = -0;         % theta target [deg]
alpha = 0;              % alpha [deg]

step = [10, 20, 30, 50];

%% step 1
if time < step(1)
    v_avanz=0;
end

%% step 2
if (time>=step(1) && time < step(2))
    alpha = (time-step(1)) * 3;
    if alpha > 20 
        alpha = 20;
    end
    alpha = -alpha;
end

%% step 3
if (time >= step(2) && time <= step(3))
    alpha = -20;
end


%% step 4
if (time >= step(3) && time <= step(4))
    alpha = 20 - (time-step(3)) * 3;
    if alpha < -20
        alpha = -20;
    end
    alpha = - alpha;
end

if time > step(4)
    alpha = (time-step(4))*3;
    if alpha > 20
        alpha = 20;
    end
end

== matlab function system2020b/Reference generator/ref 7, id 8/MATLAB Function ==
  data: time input; control_type output; v_avanz output; theta_ref output; alpha output
% Robotics project, Menolotto Mariangela & Stefano Maugeri
function [control_type, v_avanz, theta_ref, alpha] = fcn6(time)
% alpha = 0, theta=0, 1 gradino di velocità a 0.2 e un altro per fermarlo
%
speed = 1;              % speed controller
position = 2;           % return to zero controller

control_type = speed;   % could be 'speed' or 'position' 
v_avanz = 0;            % forward speed [m/s]
theta_ref = 0;         % theta target [deg]
alpha = 15;              % alpha [deg]

step = [10, 20, 30];

%% step 1
if time < step(1)
    v_avanz=0;
end

%% step 2
if (time>=step(1) && time < step(2))
    v_avanz=0.25;
end

%% step 3
if (time >= step(2) && time <= step(3))
    v_avanz = -0.25;
end

if time > step(3)
    v_avanz=0;
end

end

== matlab function system2020b/Physical system/old model/Sistema fisico1/MATLAB Function3 ==
  data: q input; B output; alpha parameter
function B = matrix_B(q, alpha)
% Robotics project, Menolotto Mariangela & Stefano Maugeri
theta = q(3);
phi = q(4);

B=B_dynamic_matrix(phi, theta);

== matlab function system2020b/Physical system/old model/Sistema fisico1/MATLAB Function7 ==
  data: q input; qdot input; C output; alpha parameter
function C = matrix_C(q, qdot, alpha)
% Robotics project, Menolotto Mariangela & Stefano Maugeri
theta = q(3);
phi = q(4);

thetadot = qdot(3);
phidot = qdot(4);

C=C_dynamic_matrix(phi,phidot,theta,thetadot);

== matlab function system2020b/Physical system/old model/Sistema fisico1/MATLAB Function8 ==
  data: q input; G output; mw parameter; mb parameter; g parameter; alpha parameter; L parameter
function G = vector_G(q, mw, mb, g, alpha, L)
% Robotics project, Menolotto Mariangela & Stefano Maugeri

theta = q(3);
phi = q(4);

G = G_dynamic_vector(alpha,phi,theta)

== matlab function system2020b/Physical system/old model/Sistema fisico1/MATLAB Function9 ==
  data: q input; S output; r parameter; l parameter
function S = matrix_S(q, r, l)
% Robotics project, Menolotto Mariangela & Stefano Maugeri
theta = q(3);

S = [-sin(theta), 0, 0;
    cos(theta), 0, 0;
    0, 1, 0;
    0, 0, 1;
    -1/r, -l/r, -1;
    -1/r, l/r, -1];

== matlab function system2020b/Reference generator/ref 9, id 10/MATLAB Function ==
  data: time input; control_type output; v_avanz output; theta output; alpha output
% Robotics project, Menolotto Mariangela & Stefano Maugeri
function [control_type, v_avanz, theta, alpha] = fcn6(time)
% alpha = 0, theta=0, 1 gradino di velocità a 0.2 e un altro per fermarlo
%
speed = 1;              % speed controller
position = 2;           % return to zero controller

control_type = speed;   % could be 'speed' or 'position' 
v_avanz = 0.0;            % forward speed [m/s]
theta = 0;         % theta target [deg]
alpha = 0;              % alpha [deg]

step = [5, 10, 20, 40];

%% step 1 0-5
if time < step(1)
    theta=0;
    v_avanz=0;
end

%% step 2 5-10
if time>=step(1) && time < step(2)
    theta = 45;
end

%% step 3 10 - 20
if time>=step(2) && time < step(3)
    theta = 45;
    alpha = (time-step(2))*1.5;
     if alpha >= 15
         alpha = 15;
     end

end

%% step 4 20 - 40
if time>=step(3) && time < step(4)
    theta = 0;
    alpha = 15;
    
end

%% step 4 40 - 50
if time >=step(4)
    v_avanz=0.25;
    alpha = 15;
end

== matlab function system2020b/Physical system/MATLAB Function3 ==
  data: q input; B output
function B = matrix_B(q)
theta = q(3);
phi = q(4);
% Robotics project, Menolotto Mariangela & Stefano Maugeri

B=B_dynamic_matrix(phi, theta);

== matlab function system2020b/Physical system/MATLAB Function5 ==
  data: M input; M_inv output
function M_inv = inverse(M)

M_inv = inv(M);

== matlab function system2020b/Reference generator/ref 3, id 4/MATLAB Function ==
  data: time input; control_type output; v_avanz output; theta_ref output; alpha output
% Robotics project, Menolotto Mariangela & Stefano Maugeri
function [control_type, v_avanz, theta_ref, alpha] = fcn3(time)
% alpha = 0, theta=0, 1 gradino di velocità a 0.2 e un altro per fermarlo
%
speed = 1;              % speed controller
position = 2;           % return to zero controller

control_type = speed;   % could be 'speed' or 'position' 
v_avanz = 0;            % forward speed [m/s]
theta_ref = 0;          % theta target [deg]
alpha = 15;              % alpha [deg]

step = [10, 20, 30];

%% step 1
if time < step(1)
    v_avanz=0;
end

%% step 2
if (time>=step(1) && time < step(2))
    
    if time > step(1) + 4
        v_avanz=0.25;
        theta_ref = -90;
    else
        theta_ref = 0;
    end
    
end

%% step 3
if (time >= step(2) && time <= step(3))
    theta_ref = -90;
    v_avanz = 0.25;
end

== matlab function system2020b/Controller/model/MATLAB Function2 ==
  data: Sr_inv output; r parameter; l parameter
function Sr_inv = matrix_S_r( r, l)
% Robotics project, Menolotto Mariangela & Stefano Maugeri


Sr_inv = inv([ -l/r, -1;
     l/r, -1]');

== matlab function system2020b/Physical system/MATLAB Function7 ==
  data: q input; qdot input; C output
function C = matrix_C(q, qdot)
% Robotics project, Menolotto Mariangela & Stefano Maugeri
theta = q(3);
phi = q(4);

thetadot = qdot(3);
phidot = qdot(4);

C=C_dynamic_matrix(phi,phidot,theta,thetadot);

== matlab function system2020b/Physical system/MATLAB Function8 ==
  data: q input; G output; alpha input
function G = vector_G(q, alpha)
% Robotics project, Menolotto Mariangela & Stefano Maugeri

theta = q(3);
phi = q(4);

G = G_dynamic_vector(alpha,phi,theta);

== matlab function system2020b/Physical system/MATLAB Function9 ==
  data: q input; S output; r parameter; l parameter
function S = matrix_S(q, r, l)
theta = q(3);
% Robotics project, Menolotto Mariangela & Stefano Maugeri

S = [-sin(theta), 0, 0;
    cos(theta), 0, 0;
    0, 1, 0;
    0, 0, 1;
    -1/r, -l/r, -1;
    -1/r, l/r, -1];

== matlab function system2020b/Physical system/S dot ==
  data: coords input; S_der output; r parameter; coordsDer input
function S_der = matrix_S_der(coords,r, coordsDer)
% Robotics project, Menolotto Mariangela & Stefano Maugeri

theta = coords(3);
thetadot = coordsDer(3);

S_der = zeros(6,3);

S_der = [-cos(theta)*thetadot, 0, 0;
    -sin(theta)*thetadot, 0, 0;
    0, 0, 0;
    0, 0, 0;
    0, 0, 0;
    0, 0, 0];

== matlab function system2020b/Controller/model/MATLAB Function3 ==
  data: angles input; B output
function B = matrix_B(angles)
% Robotics project, Menolotto Mariangela & Stefano Maugeri
%theta = q(3);
%phi = q(4);

theta = angles(2);
phi = angles(3);


B=B_dynamic_matrix(phi, theta);

== matlab function system2020b/Reference generator/ref 8, id 9/MATLAB Function1 ==
  data: time input; control_type output; v_avanz output; theta output; alpha output
% Robotics project, Menolotto Mariangela & Stefano Maugeri
function [control_type, v_avanz, theta, alpha] = fcn6(time)
% alpha = 0, theta=0, 1 gradino di velocità a 0.2 e un altro per fermarlo
%
speed = 1;              % speed controller
position = 2;           % return to zero controller

control_type = speed;   % could be 'speed' or 'position' 
v_avanz = 0;            % forward speed [m/s]
theta = 0;         % theta target [deg]
alpha = 15;              % alpha [deg]

step = [10, 25, 40, 50];

%% step 1
if time < step(1)
    theta = 0;
    v_avanz = 0;
end

%% step 2
if (time>=step(1) && time < step(2))
    v_avanz = 0.3;
    theta = (time-step(1))*30;
     if theta >= 360
         theta = 360;
     end
end

%% step 3
if (time >= step(2) && time <= step(3))
    v_avanz = 0.3;
    theta = 360 - (time-step(2))*30;
     if theta <= 0
         theta = 0;
     end
end


%% step 4
if (time >= step(3) && time <= step(4))
    v_avanz = 0;
    theta = 0;
end
%%

if time > step(4)
    v_avanz = 0;
end

== matlab function system2020b/Reference generator/ref 8, id 9/MATLAB Function2 ==
  data: time input; control_type output; v_avanz output; theta output; alpha output; x output; y output
function [control_type, v_avanz, theta, alpha,x,y] = fcn6(time)
% alpha = 0, theta=0, 1 gradino di velocità a 0.2 e un altro per fermarlo
%
speed = 1;              % speed controller
position = 2;           % return to zero controller

control_type = speed;   % could be 'speed' or 'position' 
v_avanz = 0;            % forward speed [m/s]
theta = 0;         % theta target [deg]
alpha = 15;              % alpha [deg]

metodo_di_slow = 5;

step = [10, ...
    10+(pi/2)*metodo_di_slow, ... %1/4 di circonferenza
    10+(pi)*metodo_di_slow, ...
    10+(3/2*pi)*metodo_di_slow, ...
    10+2*pi*(metodo_di_slow),...
    10+(4*pi)*metodo_di_slow]; % da qui fermo

x=0;
y=0;
A = 1;
p = 1;
q = 2;

%% step 1
if time < step(1)
    theta = 0;
    v_avanz = 0;
end

%% step 2
if (time>=step(1) && time < step(2))
    x = A*sin(p*(time-step(1)) +pi/2)-A;
    y = A*sin(q*(time-step(1)));

    xdot = -p*A*sin(p*(time-step(1)));
    ydot = q*A * cos(q*time-step(1));

    theta = (time-step(1))*(180/(step(2)-step(1)));
    if theta >= 180
        theta = 180;
    end

    v_avanz = -(-sin(theta)*xdot + cos(theta)*ydot);
end


%% step 3
if (time >= step(2) && time <= step(3))
    x = A*sin(p*(time-step(1)) +pi/2)-A;
    y = A*sin(q*(time-step(1)));

    xdot = -p*A*sin(p*(time-step(1)));
    ydot = q*A * cos(q*time-step(1));

    theta = 180 + (time-step(2))*(180/(step(2)-step(1)));
    if theta >= 360
        theta = 360;
    end
    v_avanz = -sin(theta)*xdot + cos(theta)*ydot;
end

%% step 4
if (time >= step(3) && time <= step(4))
    x = A*sin(p*(time-step(1)) +pi/2)-A;
    y = A*sin(q*(time-step(1)));

    xdot = -p*A*sin(p*(time-step(1)));
    ydot = q*A * cos(q*time-step(1));

    theta = 360 + (time-step(3))*(180/(step(2)-step(1)));
    if theta >= 540 %360+180
        theta = 540;
    end
    v_avanz = -(-sin(theta)*xdot + cos(theta)*ydot);
end

%% step 5
if (time >= step(4) && time <= step(5))
    x = A*sin(p*(time-step(1)) +pi/2)-A;
    y = A*sin(q*(time-step(1)));

    xdot = -p*A*sin(p*(time-step(1)));
    ydot = q*A * cos(q*time-step(1));

    theta = 540 + (time-step(4))*(180/(step(2)-step(1)));
    if theta >= 720
        theta = 720;
    end
    v_avanz = -sin(theta)*xdot + cos(theta)*ydot;
end

%% step 6
if time > step(5)
    v_avanz = 0;
    theta=720;
end


end

== matlab function system2020b/Controller/model/MATLAB Function7 ==
  data: angles input; nu_acc input; C output
function C = matrix_C(angles, nu_acc)
% Robotics project, Menolotto Mariangela & Stefano Maugeri
% theta = q(3);
% phi = q(4);

theta = angles(2);
phi = angles(3);

%thetadot = qdot(3);
%phidot = qdot(4);
thetadot = nu_acc(1);
phidot = nu_acc(2);

C=C_dynamic_matrix(phi,phidot,theta,thetadot);

== matlab function system2020b/Controller/model/MATLAB Function8 ==
  data: angles input; G output
function G = vector_G(angles)
% Robotics project, Menolotto Mariangela & Stefano Maugeri
% theta = q(3);
% phi = q(4);

alpha = angles(1);
theta = angles(2);
phi = angles(3);

G = G_dynamic_vector(alpha,phi,theta);

== matlab function system2020b/Controller/model/MATLAB Function9 ==
  data: angles input; S output; r parameter; l parameter
function S = matrix_S(angles, r, l)
% Robotics project, Menolotto Mariangela & Stefano Maugeri
%theta = q(3);
theta = angles(2);

S = [-sin(theta), 0, 0;
    cos(theta), 0, 0;
    0, 1, 0;
    0, 0, 1;
    -1/r, -l/r, -1;
    -1/r, l/r, -1];

== matlab function system2020b/Controller/model/S dot ==
  data: angles input; S_der output; nu_acc input
function S_der = matrix_S_der(angles, nu_acc)
% Robotics project, Menolotto Mariangela & Stefano Maugeri

%theta = coords(3);
%thetadot = coordsDer(3);
theta = angles(2);
thetadot = nu_acc(1);


S_der = zeros(6,3);

S_der = [-cos(theta)*thetadot, 0, 0;
    -sin(theta)*thetadot, 0, 0;
    0, 0, 0;
    0, 0, 0;
    0, 0, 0;
    0, 0, 0];

== matlab function system2020b/Sensors/range finder/MATLAB Function1 ==
  data: q input; d output; r parameter
function d = fcn(q, r)
% Robotics project, Menolotto Mariangela & Stefano Maugeri

phi = q(4);

a = r*(1+sin(phi));

d = a/cos(phi);
